simulink model "CentralizedWindParkModel"  (Simulink 8.2)
settings: Solver=ode45  StartTime=0.0  StopTime=inf  RelTol=1e-3
undefined symbols (not defined in the file): Take, Turbine_Library, Turbine_Profile
libraries: DDSLibrary x8
settings Model: Creator=thomas  LastModifiedBy=thomas
settings DataIOCC: SignalLoggingSaveFormat=Dataset
settings OptimizationCC: ExpressionDepthLimit=128
settings DebuggingCC: FcnCallInpInsideContextMsg=EnableAllAsError  StateNameClashWarn=none
settings GRTTargetCC: CombineOutputUpdateFcns=on  GRTInterface=off

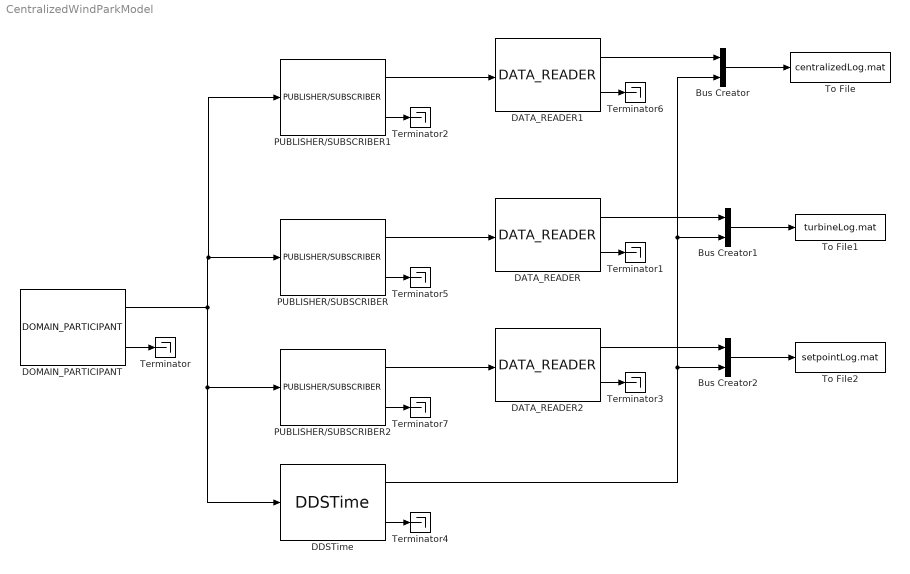
== system CentralizedWindParkModel ==
  Bus Creator : BusCreator  Inputs=2
  Bus Creator1 : BusCreator  Inputs=2
  Bus Creator2 : BusCreator  Inputs=2
  DATA_READER : DDSLibrary/DATA_READER  SFunctionSpec=)  SParam2=TurbineDataMessage  SParam3=TurbineDataReply  SParam4=-1  SParam1=on  SParam6=1  SParam7=Take()  SParam5=Turbine_Library::Turbine_Profile
  DATA_READER1 : DDSLibrary/DATA_READER  SFunctionSpec=)  SParam2=RequestMessage  SParam3=TurbineDataRequest  SParam4=-1  SParam1=on  SParam6=1  SParam7=Take()  SParam5=Turbine_Library::Turbine_Profile
  DATA_READER2 : DDSLibrary/DATA_READER  SFunctionSpec=)  SParam2=SetpointMessage  SParam3=Cluster 1  SParam4=-1  SParam1=off  SParam6=2  SParam7=Take()  SParam5=Turbine_Library::Turbine_Profile
  DDSTime : DDSLibrary/DDSTime  SFunctionSpec=[]
  DOMAIN_PARTICIPANT : DDSLibrary/DOMAIN_PARTICIPANT  SFunctionSpec=)  SParam1=-1  SParam2=Turbine_Library::Turbine_Profile  SParam3=0
  PUBLISHER/SUBSCRIBER : DDSLibrary/PUBLISHER//SUBSCRIBER  SFunctionSpec=)  SParam2=Subscriber  SParam1=-1  SParam3=Turbine_Library::Turbine_Profile
  PUBLISHER/SUBSCRIBER1 : DDSLibrary/PUBLISHER//SUBSCRIBER  SFunctionSpec=)  SParam2=Subscriber  SParam1=-1  SParam3=Turbine_Library::Turbine_Profile
  PUBLISHER/SUBSCRIBER2 : DDSLibrary/PUBLISHER//SUBSCRIBER  SFunctionSpec=)  SParam2=Subscriber  SParam1=-1  SParam3=Turbine_Library::Turbine_Profile
  Terminator{,1..7} (8 alike) : Terminator
  To File : ToFile  Filename=centralizedLog.mat  MatrixName=centralizedLog  SaveFormat=Timeseries
  To File1 : ToFile  Filename=turbineLog.mat  MatrixName=tuirbineLog  SaveFormat=Timeseries
  To File2 : ToFile  Filename=setpointLog.mat  MatrixName=setpointLog  SaveFormat=Timeseries
  wires:
  PUBLISHER/SUBSCRIBER1/1 -> DATA_READER1/1
  DATA_READER1/1 -> Bus Creator/1
  Bus Creator/1 -> To File/1
  DOMAIN_PARTICIPANT/1 -> PUBLISHER/SUBSCRIBER/1, PUBLISHER/SUBSCRIBER1/1, DDSTime/1, PUBLISHER/SUBSCRIBER2/1
  DDSTime/1 -> Bus Creator2/2, Bus Creator1/2, Bus Creator/2
  DOMAIN_PARTICIPANT/2 -> Terminator/1
  PUBLISHER/SUBSCRIBER1/2 -> Terminator2/1
  DDSTime/2 -> Terminator4/1
  DATA_READER1/2 -> Terminator6/1
  PUBLISHER/SUBSCRIBER/1 -> DATA_READER/1
  PUBLISHER/SUBSCRIBER2/1 -> DATA_READER2/1
  DATA_READER/2 -> Terminator1/1
  DATA_READER2/2 -> Terminator3/1
  DATA_READER2/1 -> Bus Creator2/1
  Bus Creator2/1 -> To File2/1
  DATA_READER/1 -> Bus Creator1/1
  Bus Creator1/1 -> To File1/1
  PUBLISHER/SUBSCRIBER/2 -> Terminator5/1
  PUBLISHER/SUBSCRIBER2/2 -> Terminator7/1
